simulink model "magnetorquerbis"  (R2019a)
settings: Solver=ode5  StartTime=0.0  StopTime=10.0  RelTol=1e-3
undefined symbols (not defined in the file or in its folder): sat
libraries: sharedutil x10, simulink x3
settings Model: Creator=Florian  LastModifiedBy=Florian

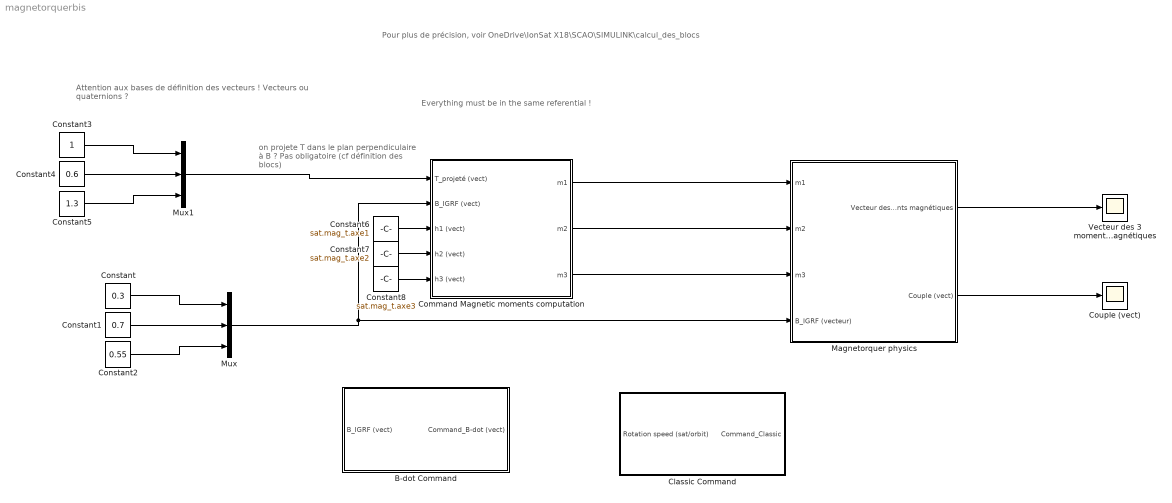
== system magnetorquerbis ==
  note: Attention aux bases de définition des vecteurs !
      |
      | Vecteurs ou quaternions ?
  note: on projete T dans
      | le plan perpendiculaire à B ?
      | Pas obligatoire (cf définition des blocs)
  note: Everything must be in the same referential !
  note: Pour plus de précision, voir OneDrive\IonSat X18\SCAO\SIMULINK\calcul_des_blocs
  B-dot Command : Subsystem
  Classic Command : Subsystem
  Command Magnetic moments computation : Subsystem
  Constant : Constant  Value=0.3
  Constant1 : Constant  Value=0.7
  Constant2 : Constant  Value=0.55
  Constant3 : Constant
  Constant4 : Constant  Value=0.6
  Constant5 : Constant  Value=1.3
  Constant6 : Constant  Value=sat.mag_t.axe1
  Constant7 : Constant  Value=sat.mag_t.axe2
  Constant8 : Constant  Value=sat.mag_t.axe3
  Couple (vect) : Scope
  Magnetorquer physics : Subsystem
  Mux : Mux  Inputs=3
  Mux1 : Mux  Inputs=3
  Vecteur des 3 moments magnétiques : Scope
  wires:
  Magnetorquer physics/1(Vecteur des 3 moments magnétiques) -> Vecteur des 3 moments magnétiques/1
  Command Magnetic moments computation/2(m2) -> Magnetorquer physics/2(m2)
  Magnetorquer physics/2(Couple (vect)) -> Couple (vect)/1
  Command Magnetic moments computation/3(m3) -> Magnetorquer physics/3(m3)
  Mux/1 -> Magnetorquer physics/4(B_IGRF (vecteur)), Command Magnetic moments computation/2(B_IGRF (vect))
  Constant/1 -> Mux/1
  Constant1/1 -> Mux/2
  Constant2/1 -> Mux/3
  Constant5/1 -> Mux1/3
  Constant4/1 -> Mux1/2
  Constant3/1 -> Mux1/1
  Mux1/1 -> Command Magnetic moments computation/1(T_projeté (vect))
  Command Magnetic moments computation/1(m1) -> Magnetorquer physics/1(m1)
  Constant6/1 -> Command Magnetic moments computation/3(h1 (vect))
  Constant7/1 -> Command Magnetic moments computation/4(h2 (vect))
  Constant8/1 -> Command Magnetic moments computation/5(h3 (vect))

== system magnetorquerbis/B-dot Command ==
  note: Dans le bras du haut, il faut entrer le champ
      | dans ref du vehicule pour la dérivation, puis remettre
      | dans le référentiel voulu
  B_IGRF (vect) : Inport
  3x3 Cross Product : sharedutil/3x3 Cross Product  aMode=aMode
      settings: SourceProductBaseCode=AE
  Derivative : Derivative
  Gain : Gain  Gain=- sat.PID.k_mag_bdot
  Command_B-dot (vect) : Outport
  wires:
  Derivative/1 -> 3x3 Cross Product/1
  Gain/1 -> Command_B-dot (vect)/1
  B_IGRF (vect)/1 -> Derivative/1, 3x3 Cross Product/2
  3x3 Cross Product/1 -> Gain/1

== system magnetorquerbis/Classic Command ==
  Rotation speed (sat/orbit) : Inport
  Gain : Gain  Gain=- sat.PID.k_mag_classic
  Command_Classic : Outport
  wires:
  Rotation speed (sat/orbit)/1 -> Gain/1
  Gain/1 -> Command_Classic/1

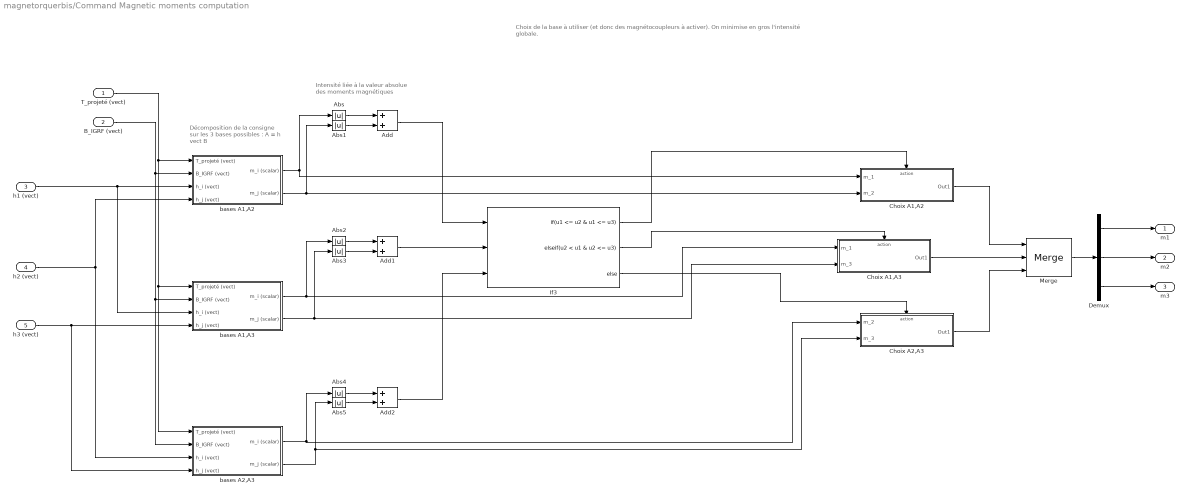
== system magnetorquerbis/Command Magnetic moments computation ==
  note: Intensité liée à la valeur absolue
      | des moments magnétiques
  note: Décomposition de la consigne
      | sur les 3 bases possibles :
      | A = h vect B
  note: Choix de la base à utiliser (et donc des magnétocoupleurs à activer). On minimise en gros l'intensité globale.
  T_projeté (vect) : Inport
  B_IGRF (vect) : Inport  Port=2
  h1 (vect) : Inport  Port=3
  h2 (vect) : Inport  Port=4
  h3 (vect) : Inport  Port=5
  Abs{,1..5} (6 alike) : Abs
  Add : Sum
  Add1 : Sum
  Add2 : Sum
  Choix A1,A2 : Subsystem  TreatAsAtomicUnit=on
  Choix A1,A3 : Subsystem  TreatAsAtomicUnit=on
  Choix A2,A3 : Subsystem  TreatAsAtomicUnit=on
  Demux : Demux  Outputs=3
  If3 : If  NumInputs=3  IfExpression=u1 <= u2 & u1 <= u3  ElseIfExpressions=u2 < u1 & u2 <= u3
  Merge : Merge  Inputs=3
  bases A1,A2 : Subsystem
  bases A1,A3 : Subsystem
  bases A2,A3 : Subsystem
  m1 : Outport
  m2 : Outport  Port=2
  m3 : Outport  Port=3
  wires:
  T_projeté (vect)/1 -> bases A2,A3/1(T_projeté (vect)), bases A1,A3/1(T_projeté (vect)), bases A1,A2/1(T_projeté (vect))
  B_IGRF (vect)/1 -> bases A2,A3/2(B_IGRF (vect)), bases A1,A3/2(B_IGRF (vect)), bases A1,A2/2(B_IGRF (vect))
  h1 (vect)/1 -> bases A1,A3/3(h_i (vect)), bases A1,A2/3(h_i (vect))
  h2 (vect)/1 -> bases A2,A3/3(h_i (vect)), bases A1,A2/4(h_j (vect))
  h3 (vect)/1 -> bases A2,A3/4(h_j (vect)), bases A1,A3/4(h_j (vect))
  Abs/1 -> Add/1
  bases A1,A2/1(m_i (scalar)) -> Choix A1,A2/1(m_1), Abs/1
  bases A1,A2/2(m_j (scalar)) -> Abs1/1, Choix A1,A2/2(m_2)
  Abs1/1 -> Add/2
  Abs3/1 -> Add1/2
  Abs2/1 -> Add1/1
  Abs5/1 -> Add2/2
  Abs4/1 -> Add2/1
  bases A1,A3/1(m_i (scalar)) -> Choix A1,A3/1(m_1), Abs2/1
  bases A1,A3/2(m_j (scalar)) -> Choix A1,A3/2(m_3), Abs3/1
  bases A2,A3/2(m_j (scalar)) -> Abs5/1, Choix A2,A3/2(m_3)
  Choix A1,A2/1(Out1) -> Merge/1
  Choix A1,A3/1(Out1) -> Merge/2
  Demux/3 -> m3/1
  Demux/2 -> m2/1
  Demux/1 -> m1/1
  Add/1 -> If3/1
  Add1/1 -> If3/2
  Add2/1 -> If3/3
  If3/1 -> Choix A1,A2/Action
  If3/2 -> Choix A1,A3/Action
  If3/3 -> Choix A2,A3/Action
  Choix A2,A3/1(Out1) -> Merge/3
  bases A2,A3/1(m_i (scalar)) -> Abs4/1, Choix A2,A3/1(m_2)
  Merge/1 -> Demux/1

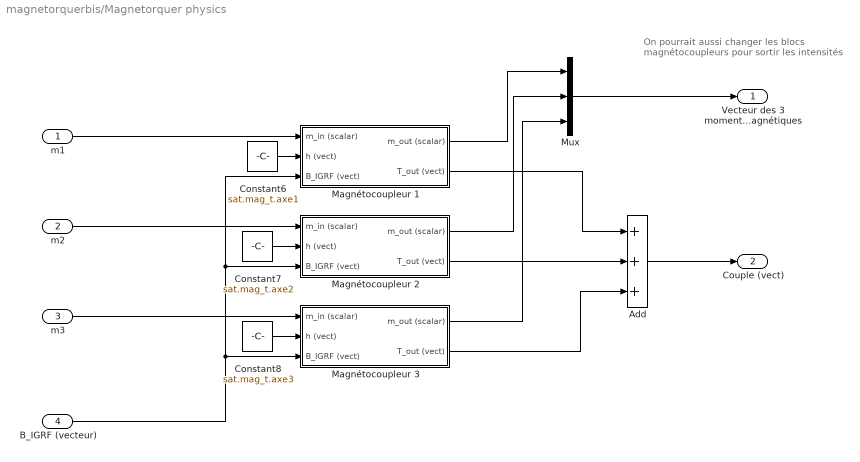
== system magnetorquerbis/Magnetorquer physics ==
  note: On pourrait aussi changer les blocs
      | magnétocoupleurs pour sortir les intensités
  m1 : Inport
  m2 : Inport  Port=2
  m3 : Inport  Port=3
  B_IGRF (vecteur) : Inport  Port=4
  Add : Sum  Inputs=+++
  Constant6 : Constant  Value=sat.mag_t.axe1
  Constant7 : Constant  Value=sat.mag_t.axe2
  Constant8 : Constant  Value=sat.mag_t.axe3
  Magnétocoupleur 1 : Subsystem
  Magnétocoupleur 2 : Subsystem
  Magnétocoupleur 3 : Subsystem
  Mux : Mux  Inputs=3
  Vecteur des 3 moments magnétiques : Outport
  Couple (vect) : Outport  Port=2
  wires:
  Constant6/1 -> Magnétocoupleur 1/2(h (vect))
  B_IGRF (vecteur)/1 -> Magnétocoupleur 1/3(B_IGRF (vect)), Magnétocoupleur 2/3(B_IGRF (vect)), Magnétocoupleur 3/3(B_IGRF (vect))
  Constant7/1 -> Magnétocoupleur 2/2(h (vect))
  Magnétocoupleur 2/1(m_out (scalar)) -> Mux/2
  Add/1 -> Couple (vect)/1
  Magnétocoupleur 1/2(T_out (vect)) -> Add/1
  Magnétocoupleur 2/2(T_out (vect)) -> Add/2
  Magnétocoupleur 3/2(T_out (vect)) -> Add/3
  Mux/1 -> Vecteur des 3 moments magnétiques/1
  m3/1 -> Magnétocoupleur 3/1(m_in (scalar))
  Magnétocoupleur 1/1(m_out (scalar)) -> Mux/1
  Magnétocoupleur 3/1(m_out (scalar)) -> Mux/3
  m2/1 -> Magnétocoupleur 2/1(m_in (scalar))
  Constant8/1 -> Magnétocoupleur 3/2(h (vect))
  m1/1 -> Magnétocoupleur 1/1(m_in (scalar))

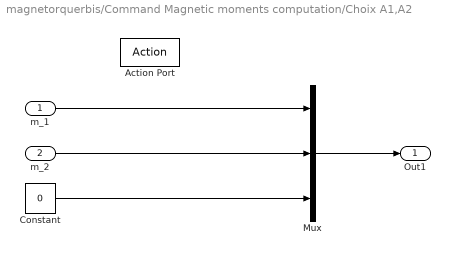
== system magnetorquerbis/Command Magnetic moments computation/Choix A1,A2 ==
  m_1 : Inport
  m_2 : Inport  Port=2
  Action Port : ActionPort  ActionPortLabel=if(u1 <= u2 & u1 <= u3)
  Constant : Constant  Value=0
  Mux : Mux  Inputs=3
  Out1 : Outport
  wires:
  m_1/1 -> Mux/1
  m_2/1 -> Mux/2
  Constant/1 -> Mux/3
  Mux/1 -> Out1/1

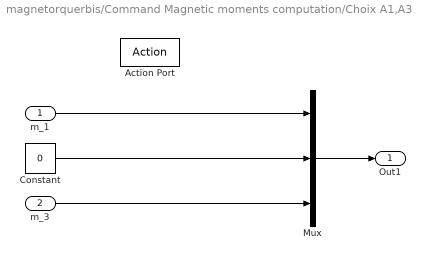
== system magnetorquerbis/Command Magnetic moments computation/Choix A1,A3 ==
  m_1 : Inport
  m_3 : Inport  Port=2
  Action Port : ActionPort  ActionPortLabel=elseif(u2 < u1 & u2 <= u3)
  Constant : Constant  Value=0
  Mux : Mux  Inputs=3
  Out1 : Outport
  wires:
  m_1/1 -> Mux/1
  m_3/1 -> Mux/3
  Constant/1 -> Mux/2
  Mux/1 -> Out1/1

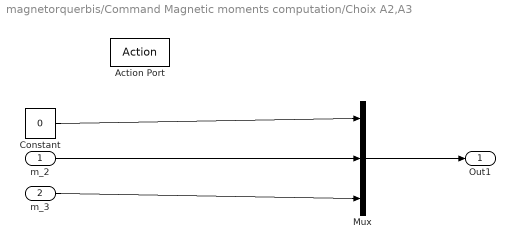
== system magnetorquerbis/Command Magnetic moments computation/Choix A2,A3 ==
  m_2 : Inport
  m_3 : Inport  Port=2
  Action Port : ActionPort  ActionPortLabel=else
  Constant : Constant  Value=0
  Mux : Mux  Inputs=3
  Out1 : Outport
  wires:
  m_2/1 -> Mux/2
  m_3/1 -> Mux/3
  Constant/1 -> Mux/1
  Mux/1 -> Out1/1

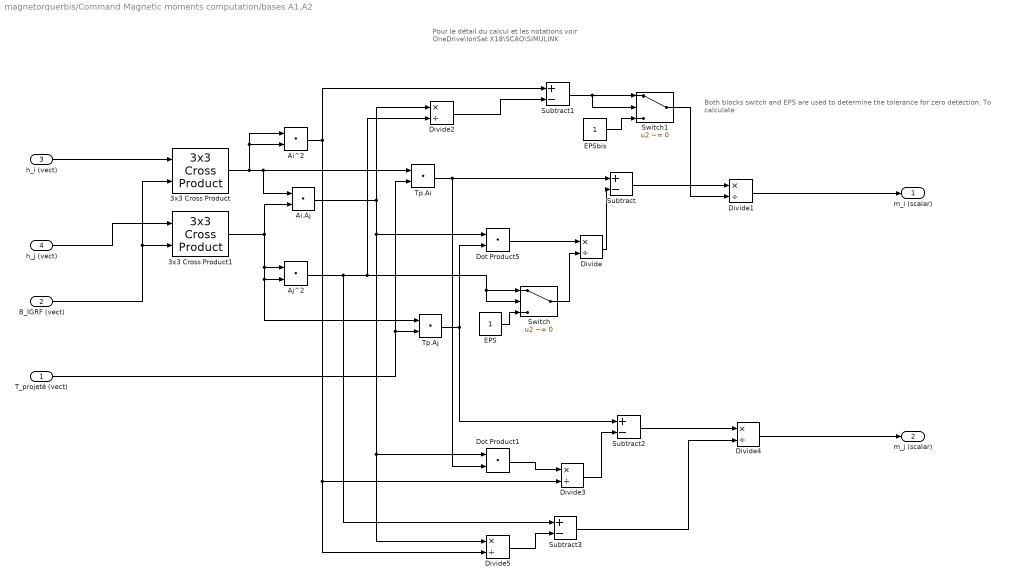
== system magnetorquerbis/Command Magnetic moments computation/bases A1,A2 ==
  note: Both blocks switch and EPS are used to determine the tolerance for zero detection.
      | To calculate
  note: Pour le détail du calcul et les notations voir
      | OneDrive\IonSat X18\SCAO\SIMULINK
  T_projeté (vect) : Inport
  B_IGRF (vect) : Inport  Port=2
  h_i (vect) : Inport  Port=3
  h_j (vect) : Inport  Port=4
  3x3 Cross Product : sharedutil/3x3 Cross Product  aMode=aMode
      settings: SourceProductBaseCode=AE
  3x3 Cross Product1 : sharedutil/3x3 Cross Product  aMode=aMode
      settings: SourceProductBaseCode=AE
  Ai.Aj : DotProduct  InputSameDT=on  OutDataTypeStr=Inherit: Inherit via internal rule
  Ai^2 : DotProduct  InputSameDT=on  OutDataTypeStr=Inherit: Inherit via internal rule
  Aj^2 : DotProduct  InputSameDT=on  OutDataTypeStr=Inherit: Inherit via internal rule
  Divide{,1..5} (6 alike) : Product  Inputs=*/
  Dot Product1 : DotProduct  InputSameDT=on  OutDataTypeStr=Inherit: Inherit via internal rule
  Dot Product5 : DotProduct  InputSameDT=on  OutDataTypeStr=Inherit: Inherit via internal rule
  EPS : Constant
  EPSbis : Constant
  Subtract{,1..3} (4 alike) : Sum  Inputs=+-
  Switch : Switch  Criteria=u2 ~= 0
  Switch1 : Switch  Criteria=u2 ~= 0
  Tp.Ai : DotProduct  InputSameDT=on  OutDataTypeStr=Inherit: Inherit via internal rule
  Tp.Aj : DotProduct  InputSameDT=on  OutDataTypeStr=Inherit: Inherit via internal rule
  m_i (scalar) : Outport
  m_j (scalar) : Outport  Port=2
  wires:
  h_j (vect)/1 -> 3x3 Cross Product1/1
  h_i (vect)/1 -> 3x3 Cross Product/1
  B_IGRF (vect)/1 -> 3x3 Cross Product/2, 3x3 Cross Product1/2
  3x3 Cross Product/1 -> Ai.Aj/1, Tp.Ai/1, Ai^2/1, Ai^2/2
  3x3 Cross Product1/1 -> Ai.Aj/2, Tp.Aj/1, Aj^2/2, Aj^2/1
  T_projeté (vect)/1 -> Tp.Aj/2, Tp.Ai/2
  Tp.Ai/1 -> Dot Product1/2, Subtract/1
  Ai.Aj/1 -> Divide5/1, Dot Product1/1, Dot Product5/1, Divide2/1
  Tp.Aj/1 -> Subtract2/1, Dot Product5/2
  Aj^2/1 -> Subtract3/1, Switch/2, Switch/1, Divide2/2
  Dot Product5/1 -> Divide/1
  Divide/1 -> Subtract/2
  Subtract/1 -> Divide1/1
  Ai^2/1 -> Divide5/2, Divide3/2, Subtract1/1
  Subtract1/1 -> Switch1/2, Switch1/1
  Divide2/1 -> Subtract1/2
  Divide1/1 -> m_i (scalar)/1
  Dot Product1/1 -> Divide3/1
  Divide3/1 -> Subtract2/2
  Subtract2/1 -> Divide4/1
  Divide5/1 -> Subtract3/2
  Subtract3/1 -> Divide4/2
  Divide4/1 -> m_j (scalar)/1
  EPS/1 -> Switch/3
  Switch/1 -> Divide/2
  EPSbis/1 -> Switch1/3
  Switch1/1 -> Divide1/2

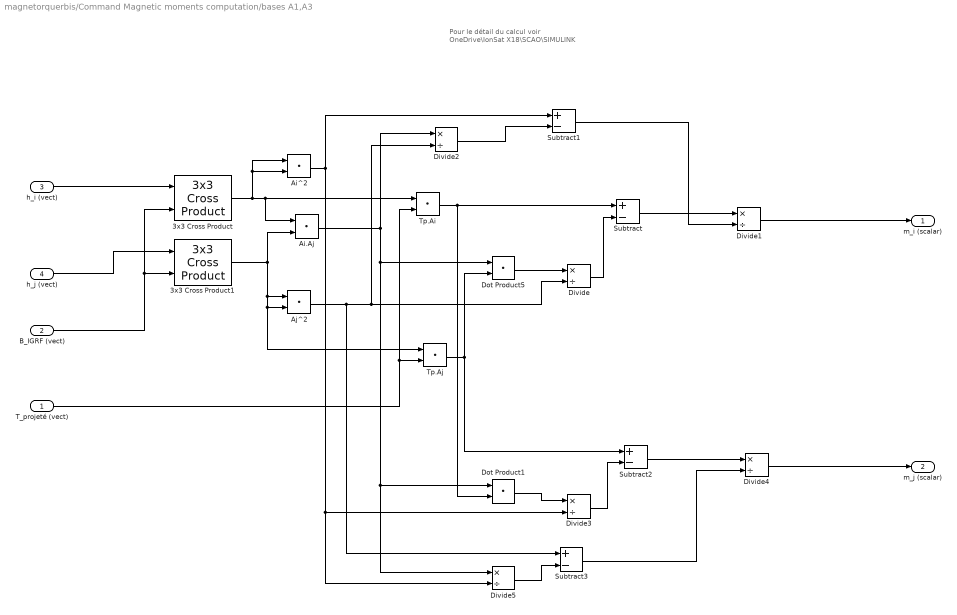
== system magnetorquerbis/Command Magnetic moments computation/bases A1,A3 ==
  note: Pour le détail du calcul voir
      | OneDrive\IonSat X18\SCAO\SIMULINK
  T_projeté (vect) : Inport
  B_IGRF (vect) : Inport  Port=2
  h_i (vect) : Inport  Port=3
  h_j (vect) : Inport  Port=4
  3x3 Cross Product : sharedutil/3x3 Cross Product  aMode=aMode
      settings: SourceProductBaseCode=AE
  3x3 Cross Product1 : sharedutil/3x3 Cross Product  aMode=aMode
      settings: SourceProductBaseCode=AE
  Ai.Aj : DotProduct  InputSameDT=on  OutDataTypeStr=Inherit: Inherit via internal rule
  Ai^2 : DotProduct  InputSameDT=on  OutDataTypeStr=Inherit: Inherit via internal rule
  Aj^2 : DotProduct  InputSameDT=on  OutDataTypeStr=Inherit: Inherit via internal rule
  Divide{,1..5} (6 alike) : Product  Inputs=*/
  Dot Product1 : DotProduct  InputSameDT=on  OutDataTypeStr=Inherit: Inherit via internal rule
  Dot Product5 : DotProduct  InputSameDT=on  OutDataTypeStr=Inherit: Inherit via internal rule
  Subtract{,1..3} (4 alike) : Sum  Inputs=+-
  Tp.Ai : DotProduct  InputSameDT=on  OutDataTypeStr=Inherit: Inherit via internal rule
  Tp.Aj : DotProduct  InputSameDT=on  OutDataTypeStr=Inherit: Inherit via internal rule
  m_i (scalar) : Outport
  m_j (scalar) : Outport  Port=2
  wires:
  h_j (vect)/1 -> 3x3 Cross Product1/1
  h_i (vect)/1 -> 3x3 Cross Product/1
  B_IGRF (vect)/1 -> 3x3 Cross Product/2, 3x3 Cross Product1/2
  3x3 Cross Product/1 -> Ai.Aj/1, Tp.Ai/1, Ai^2/1, Ai^2/2
  3x3 Cross Product1/1 -> Ai.Aj/2, Tp.Aj/1, Aj^2/2, Aj^2/1
  T_projeté (vect)/1 -> Tp.Aj/2, Tp.Ai/2
  Tp.Ai/1 -> Dot Product1/2, Subtract/1
  Ai.Aj/1 -> Divide5/1, Dot Product1/1, Dot Product5/1, Divide2/1
  Tp.Aj/1 -> Subtract2/1, Dot Product5/2
  Aj^2/1 -> Subtract3/1, Divide2/2, Divide/2
  Dot Product5/1 -> Divide/1
  Divide/1 -> Subtract/2
  Subtract/1 -> Divide1/1
  Ai^2/1 -> Divide5/2, Divide3/2, Subtract1/1
  Subtract1/1 -> Divide1/2
  Divide2/1 -> Subtract1/2
  Divide1/1 -> m_i (scalar)/1
  Dot Product1/1 -> Divide3/1
  Divide3/1 -> Subtract2/2
  Subtract2/1 -> Divide4/1
  Divide5/1 -> Subtract3/2
  Subtract3/1 -> Divide4/2
  Divide4/1 -> m_j (scalar)/1

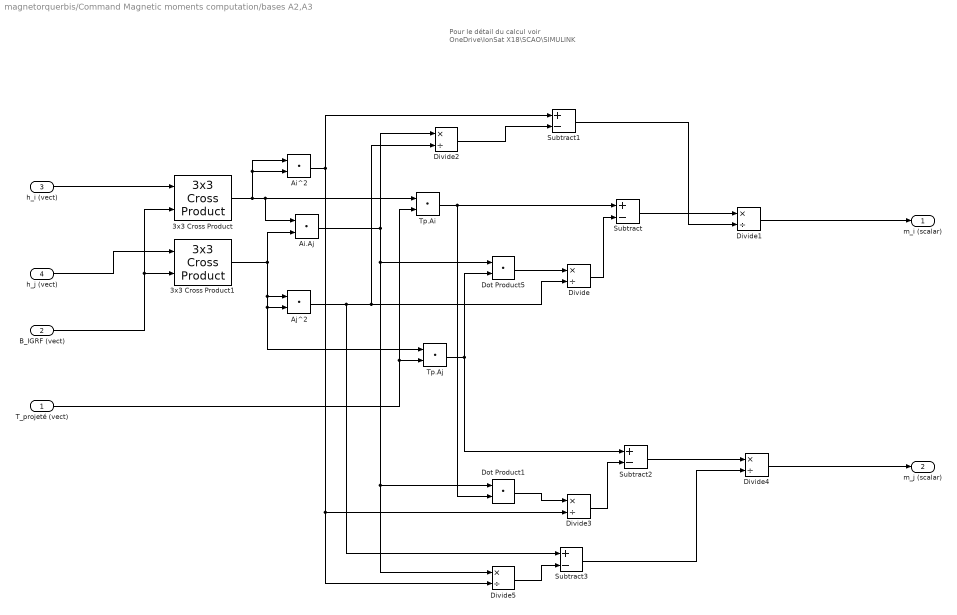
== system magnetorquerbis/Command Magnetic moments computation/bases A2,A3 ==
  note: Pour le détail du calcul voir
      | OneDrive\IonSat X18\SCAO\SIMULINK
  T_projeté (vect) : Inport
  B_IGRF (vect) : Inport  Port=2
  h_i (vect) : Inport  Port=3
  h_j (vect) : Inport  Port=4
  3x3 Cross Product : sharedutil/3x3 Cross Product  aMode=aMode
      settings: SourceProductBaseCode=AE
  3x3 Cross Product1 : sharedutil/3x3 Cross Product  aMode=aMode
      settings: SourceProductBaseCode=AE
  Ai.Aj : DotProduct  InputSameDT=on  OutDataTypeStr=Inherit: Inherit via internal rule
  Ai^2 : DotProduct  InputSameDT=on  OutDataTypeStr=Inherit: Inherit via internal rule
  Aj^2 : DotProduct  InputSameDT=on  OutDataTypeStr=Inherit: Inherit via internal rule
  Divide{,1..5} (6 alike) : Product  Inputs=*/
  Dot Product1 : DotProduct  InputSameDT=on  OutDataTypeStr=Inherit: Inherit via internal rule
  Dot Product5 : DotProduct  InputSameDT=on  OutDataTypeStr=Inherit: Inherit via internal rule
  Subtract{,1..3} (4 alike) : Sum  Inputs=+-
  Tp.Ai : DotProduct  InputSameDT=on  OutDataTypeStr=Inherit: Inherit via internal rule
  Tp.Aj : DotProduct  InputSameDT=on  OutDataTypeStr=Inherit: Inherit via internal rule
  m_i (scalar) : Outport
  m_j (scalar) : Outport  Port=2
  wires:
  h_j (vect)/1 -> 3x3 Cross Product1/1
  h_i (vect)/1 -> 3x3 Cross Product/1
  B_IGRF (vect)/1 -> 3x3 Cross Product/2, 3x3 Cross Product1/2
  3x3 Cross Product/1 -> Ai.Aj/1, Tp.Ai/1, Ai^2/1, Ai^2/2
  3x3 Cross Product1/1 -> Ai.Aj/2, Tp.Aj/1, Aj^2/2, Aj^2/1
  T_projeté (vect)/1 -> Tp.Aj/2, Tp.Ai/2
  Tp.Ai/1 -> Dot Product1/2, Subtract/1
  Ai.Aj/1 -> Divide5/1, Dot Product1/1, Dot Product5/1, Divide2/1
  Tp.Aj/1 -> Subtract2/1, Dot Product5/2
  Aj^2/1 -> Subtract3/1, Divide2/2, Divide/2
  Dot Product5/1 -> Divide/1
  Divide/1 -> Subtract/2
  Subtract/1 -> Divide1/1
  Ai^2/1 -> Divide5/2, Divide3/2, Subtract1/1
  Divide2/1 -> Subtract1/2
  Divide1/1 -> m_i (scalar)/1
  Dot Product1/1 -> Divide3/1
  Divide3/1 -> Subtract2/2
  Subtract2/1 -> Divide4/1
  Divide5/1 -> Subtract3/2
  Subtract3/1 -> Divide4/2
  Divide4/1 -> m_j (scalar)/1
  Subtract1/1 -> Divide1/2

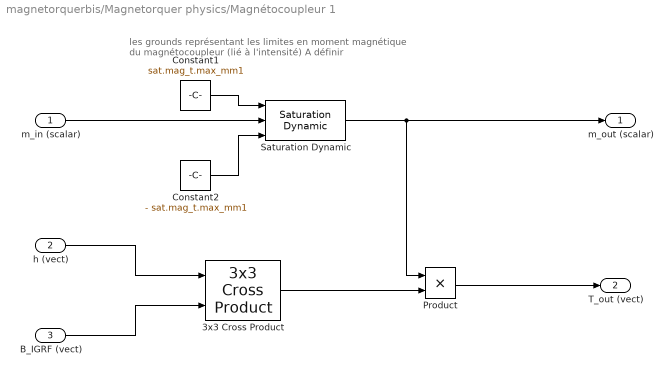
== system magnetorquerbis/Magnetorquer physics/Magnétocoupleur 1 ==
  note: les grounds représentant les limites en
      |  moment magnétique du magnétocoupleur (lié à l'intensité)
      | A définir
  m_in (scalar) : Inport
  h (vect) : Inport  Port=2
  B_IGRF (vect) : Inport  Port=3
  3x3 Cross Product : sharedutil/3x3 Cross Product  aMode=aMode
      settings: SourceProductBaseCode=AE
  Constant1 : Constant  Value=sat.mag_t.max_mm1
  Constant2 : Constant  Value=- sat.mag_t.max_mm1
  Product : Product
  Saturation Dynamic : simulink/Discontinuities/Saturation Dynamic  OutMin=[]  OutMax=[]  OutDataTypeStr=Inherit: Same as second input  OutDataType=fixdt(1, 16)  OutScaling=2^-10  DoSatur=off
  m_out (scalar) : Outport
  T_out (vect) : Outport  Port=2
  wires:
  h (vect)/1 -> 3x3 Cross Product/1
  B_IGRF (vect)/1 -> 3x3 Cross Product/2
  m_in (scalar)/1 -> Saturation Dynamic/2
  Constant2/1 -> Saturation Dynamic/3
  Constant1/1 -> Saturation Dynamic/1
  Saturation Dynamic/1 -> Product/1, m_out (scalar)/1
  3x3 Cross Product/1 -> Product/2
  Product/1 -> T_out (vect)/1

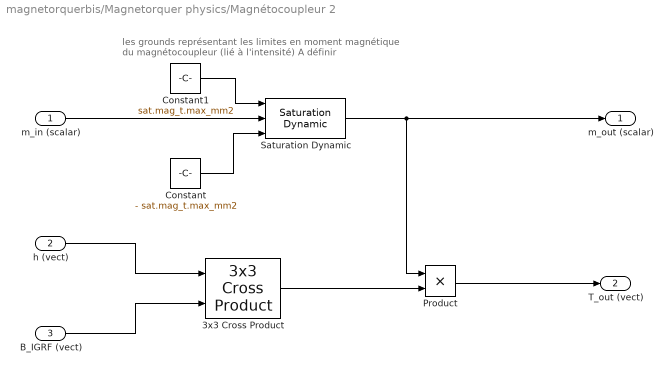
== system magnetorquerbis/Magnetorquer physics/Magnétocoupleur 2 ==
  note: les grounds représentant les limites en
      |  moment magnétique du magnétocoupleur (lié à l'intensité)
      | A définir
  m_in (scalar) : Inport
  h (vect) : Inport  Port=2
  B_IGRF (vect) : Inport  Port=3
  3x3 Cross Product : sharedutil/3x3 Cross Product  aMode=aMode
      settings: SourceProductBaseCode=AE
  Constant : Constant  Value=- sat.mag_t.max_mm2
  Constant1 : Constant  Value=sat.mag_t.max_mm2
  Product : Product
  Saturation Dynamic : simulink/Discontinuities/Saturation Dynamic  OutMin=[]  OutMax=[]  OutDataTypeStr=Inherit: Same as second input  OutDataType=fixdt(1, 16)  OutScaling=2^-10  DoSatur=off
  m_out (scalar) : Outport
  T_out (vect) : Outport  Port=2
  wires:
  h (vect)/1 -> 3x3 Cross Product/1
  B_IGRF (vect)/1 -> 3x3 Cross Product/2
  m_in (scalar)/1 -> Saturation Dynamic/2
  Constant/1 -> Saturation Dynamic/3
  Constant1/1 -> Saturation Dynamic/1
  Saturation Dynamic/1 -> Product/1, m_out (scalar)/1
  3x3 Cross Product/1 -> Product/2
  Product/1 -> T_out (vect)/1

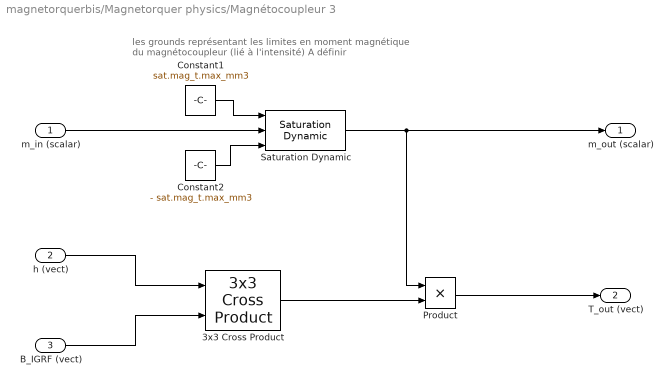
== system magnetorquerbis/Magnetorquer physics/Magnétocoupleur 3 ==
  note: les grounds représentant les limites en
      |  moment magnétique du magnétocoupleur (lié à l'intensité)
      | A définir
  m_in (scalar) : Inport
  h (vect) : Inport  Port=2
  B_IGRF (vect) : Inport  Port=3
  3x3 Cross Product : sharedutil/3x3 Cross Product  aMode=aMode
      settings: SourceProductBaseCode=AE
  Constant1 : Constant  Value=sat.mag_t.max_mm3
  Constant2 : Constant  Value=- sat.mag_t.max_mm3
  Product : Product
  Saturation Dynamic : simulink/Discontinuities/Saturation Dynamic  OutMin=[]  OutMax=[]  OutDataTypeStr=Inherit: Same as second input  OutDataType=fixdt(1, 16)  OutScaling=2^-10  DoSatur=off
  m_out (scalar) : Outport
  T_out (vect) : Outport  Port=2
  wires:
  h (vect)/1 -> 3x3 Cross Product/1
  B_IGRF (vect)/1 -> 3x3 Cross Product/2
  m_in (scalar)/1 -> Saturation Dynamic/2
  Constant2/1 -> Saturation Dynamic/3
  Constant1/1 -> Saturation Dynamic/1
  Saturation Dynamic/1 -> Product/1, m_out (scalar)/1
  3x3 Cross Product/1 -> Product/2
  Product/1 -> T_out (vect)/1
